simulink model "SimPrac6"  (R2018a)
settings: Solver=ode45  StartTime=0.0  StopTime=20  RelTol=1e-9
undefined symbols (not defined in the file): K2, K3, Kg, Kr, Ku, Kusil, M0, Mn, T1, T1g, T2, Ta, Ung
settings Model: Creator=dirlak  LastModifiedBy=dirlak

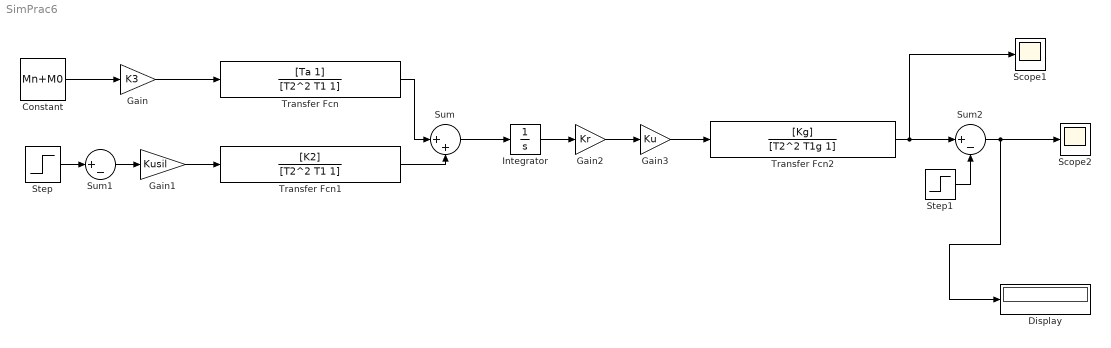
== system SimPrac6 ==
  Constant : Constant  Value=Mn+M0
  Display : Display
  Gain : Gain  Gain=K3
  Gain1 : Gain  Gain=Kusil
  Gain2 : Gain  Gain=Kr
  Gain3 : Gain  Gain=Ku
  Integrator : Integrator
  Scope1 : Scope
  Scope2 : Scope
  Step : Step  Time=0  After=Ung  SampleTime=0
  Step1 : Step  Time=15  After=Ung*0.1  SampleTime=0
  Sum : Sum  Inputs=|++
  Sum1 : Sum  Inputs=|+-
  Sum2 : Sum  Inputs=|+-
  Transfer Fcn : TransferFcn  Numerator=[Ta 1]  Denominator=[T2^2 T1 1]
  Transfer Fcn1 : TransferFcn  Numerator=[K2]  Denominator=[T2^2 T1 1]
  Transfer Fcn2 : TransferFcn  Numerator=[Kg]  Denominator=[T2^2 T1g 1]
  wires:
  Constant/1 -> Gain/1
  Gain/1 -> Transfer Fcn/1
  Transfer Fcn/1 -> Sum/1
  Transfer Fcn1/1 -> Sum/2
  Step/1 -> Sum1/1
  Sum1/1 -> Gain1/1
  Gain1/1 -> Transfer Fcn1/1
  Sum/1 -> Integrator/1
  Integrator/1 -> Gain2/1
  Gain2/1 -> Gain3/1
  Gain3/1 -> Transfer Fcn2/1
  Transfer Fcn2/1 -> Sum2/1, Scope1/1
  Sum2/1 -> Scope2/1, Display/1
  Step1/1 -> Sum2/2
